simulink model "Single_phase_input_in_sine_Wave"  (R2021a)
settings: Solver=VariableStepAuto  StartTime=0.0  StopTime=1  RelTol=1e-3
undefined symbols (not defined in the file): Ion, Lithium
libraries: spsDiodeLib x8, spsVoltageMeasurementLib x7, spsSeriesRLCBranchLib x6, spsCurrentMeasurementLib x6, spsMosfetLib x4, spsACVoltageSourceLib x1, spsBatteryLib x1, spsImpedanceMeasurementLib x1, spsMutualInductanceLib x1, simulink x1, spspowerguiLib x1
settings Model: Creator=HP  LastModifiedBy=ADMIN

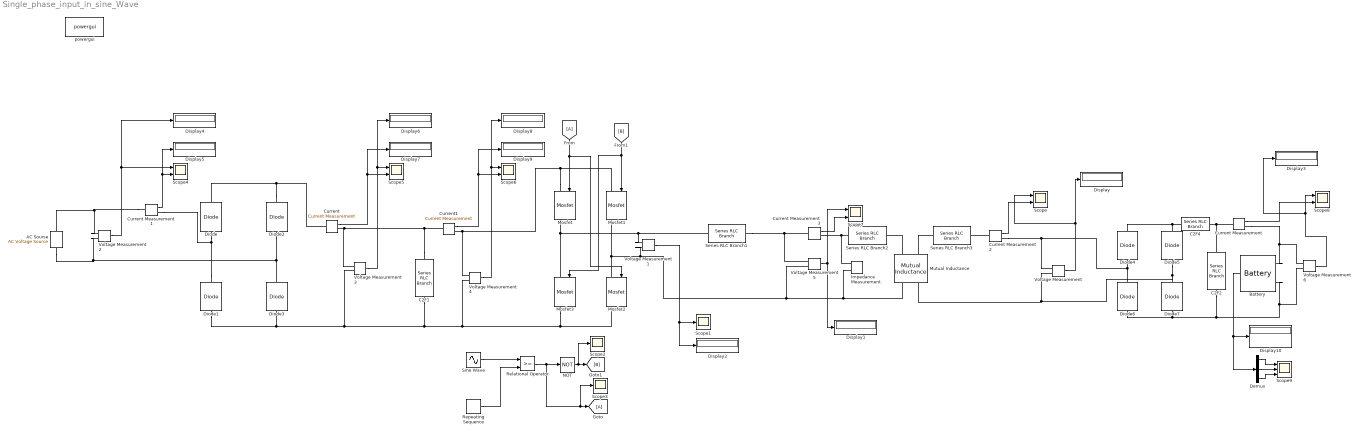
== system Single_phase_input_in_sine_Wave ==
  AC Sourse : spsACVoltageSourceLib/AC Voltage Source  Amplitude=325  Phase=0  Frequency=50  SampleTime=0  Measurements=Voltage  BusType=swing  Pref=10e3  Qref=0  Qmin=-inf  Qmax=+inf
  Battery : spsBatteryLib/Battery  BatType=Lithium-Ion  ShowTempParam=off  ThermalPreset=no  ShowAgeParam=off  NomV=240  NomQ=1  SOC=50  Batt_Tr=30  PresetModel=on  MaxQ=1  MinV=180  FullV=279.3569  Dis_rate=0.43478  R=2.4  Normal_OP=0.90435  expZone="[259.2926    0.04913043]"  current=[6.5 13 32.5]  Units=Time  Tci=20  NomT=20  T2=-30  MaxQ2=4.8  FullV2=7.1  Normal_OP2=5.655  expZone2="[6.58           1]"  Rca=0.6  ti=2000  Dp=0  Neq0=0  Tsim=1e6  Ta1=25  Qeol=5.4*0.9  Reol=0.013333*1.2  Char_age=[2.3478, 3]  Dis_age=[2.3478, 10]  N1=1500  N2=10500  N3=1000  N4=1400  Ta2=45  N5=950
  C2F1 : spsSeriesRLCBranchLib/Series RLC Branch  LConnTagsString=__new0  RConnTagsString=__new0  BranchType=C  Resistance=1e-6  Inductance=1e-3  SetiL0=off  InitialCurrent=0  Capacitance=300e-5  Setx0=off  InitialVoltage=0  Measurements=None
  C2F2 : spsSeriesRLCBranchLib/Series RLC Branch  LConnTagsString=__new0  RConnTagsString=__new0  BranchType=C  Resistance=1e-6  Inductance=1e-3  SetiL0=off  InitialCurrent=0  Capacitance=5e-6  Setx0=off  InitialVoltage=0  Measurements=None
  C2F4 : spsSeriesRLCBranchLib/Series RLC Branch  LConnTagsString=__new0  RConnTagsString=__new0  BranchType=L  Resistance=1e-6  Inductance=1e-6  SetiL0=off  InitialCurrent=0  Capacitance=5e-6  Setx0=off  InitialVoltage=0  Measurements=None
  Current : spsCurrentMeasurementLib/Current Measurement  PhasorSimulation=off  OutputType=Complex  PSBequivalent=0
  Current Measurement{,1..3} (4 alike) : spsCurrentMeasurementLib/Current Measurement  PhasorSimulation=off  OutputType=Complex  PSBequivalent=0
  Current1 : spsCurrentMeasurementLib/Current Measurement  PhasorSimulation=off  OutputType=Complex  PSBequivalent=0
  Demux : Demux  Outputs=3
  Diode{,1..7} (8 alike) : spsDiodeLib/Diode  Ron=0.001  Lon=0  Vf=0.8  IC=0  UseSnubber=0  Rs=500  Cs=250e-9  Measurements=off
  Display{,1..10} (11 alike) : Display
  Impedance Measurement : spsImpedanceMeasurementLib/Impedance Measurement  LConnTagsString=+|-  Factor=1
      settings: SourceProductBaseCode=PS
  Mosfet{,1..3} (4 alike) : spsMosfetLib/Mosfet  Ron=0.1  Lon=0  Rd=0.01  Vfd=0  IC=0  Rs=1e5  Cs=inf  Measurements=on
  Mutual Inductance : spsMutualInductanceLib/Mutual Inductance  LConnTagsString=a|b  RConnTagsString=A|B  TypeOfMutual=Two or three windings with equal mutual terms  NumberOfWindings=3  SelfImpedance1=[0.0714 73.43e-06]  SelfImpedance2=[0.0714 73.43e-06]  ThreeWindings=off  SelfImpedance3=[ 1.1 1.1e-03]  MutualImpedance=[0.01428 14.86e-06]  InductanceMatrix="[1.0 0.9  0.9 ;  0.9 1.0  0.9;  0.9 0.9 1.0 ] * 1e-3"  ResistanceMatrix="[1.0 0.9  0.9 ;  0.9 1.0  0.9;  0.9 0.9 1.0 ]"  Measurements=None
      settings: SourceProductBaseCode=PS
  NOT : Logic  Operator=NOT  IconShape=distinctive  AllPortsSameDT=off  OutDataTypeStr=boolean
  Relational Operator : RelationalOperator  OutDataTypeStr=boolean  RndMeth=Simplest
  Repeating Sequence : simulink/Sources/Repeating Sequence  rep_seq_t=[0 0.0000005 0.000001]  rep_seq_y=[-1 1 -1]
  Scope{,4..8} (6 alike) : Scope  NumInputPorts=2
  Scope1 : Scope
  Scope2 : Scope
  Scope3 : Scope
  Scope9 : Scope  NumInputPorts=3
  Series RLC Branch1 : spsSeriesRLCBranchLib/Series RLC Branch  LConnTagsString=__new0  RConnTagsString=__new0  BranchType=R  Resistance=2  Inductance=1e-3  SetiL0=off  InitialCurrent=0  Capacitance=34.5e-9  Setx0=off  InitialVoltage=0  Measurements=None
  Series RLC Branch2 : spsSeriesRLCBranchLib/Series RLC Branch  LConnTagsString=__new0  RConnTagsString=__new0  BranchType=C  Resistance=1  Inductance=1e-3  SetiL0=off  InitialCurrent=0  Capacitance=34.5e-9  Setx0=off  InitialVoltage=0  Measurements=None
  Series RLC Branch3 : spsSeriesRLCBranchLib/Series RLC Branch  LConnTagsString=__new0  RConnTagsString=__new0  BranchType=C  Resistance=1  Inductance=1e-3  SetiL0=off  InitialCurrent=0  Capacitance=34.5e-9  Setx0=off  InitialVoltage=0  Measurements=None
  Sine Wave : Sin  Amplitude=0.45  Frequency=2*pi*100000  SampleTime=0
  Voltage Measurement{,1..6} (7 alike) : spsVoltageMeasurementLib/Voltage Measurement  PhasorSimulation=off  OutputType=Complex  PSBequivalent=0
  powergui : spspowerguiLib/powergui  Priority=1  SimulationMode=Continuous  SampleTime=5e-7  frequency=60  Iterations=50  frequencyindice=0  Pbase=100e6  ErrMax=1e-4  UnitsV=kV  UnitsW=MW  buscounter=0  FunctionMessages=off  echomessages=off  EnableUseOfTLC=off  CurrentSourceSwitches=off  DisableSnubberDevices=off  DisableRonSwitches=off  DisableVfSwitches=off  DisplayEquations=off  AutomaticDiscreteSolvers=off  SolverType=Tustin/Backward Euler (TBE)  Interpol=off  ExternalGateDelay=off  methode=off  Ts=100  x0status=blocks  SPID=on  SwTol=0  HookPort=off  NonlinearTolerance=1e-4  nMaxIteration=100  ContinueOnMaxIteration=off  RestoreLinks=warning  ResistiveCurrentMeasurement=off  Frange=[0:2:1100000]  Ylog=on  Xlog=off  ShowGrid=off  save=off  variable=ZData  structure=0  ZoomFFT=off  StartTime=0.0  cycles=1  DisplayStyle=1  fundamental=60  FreqAxis=off  MaxFrequency=1000  frequencyindicesteady=1  RmsSteady=1  display=off
  wires:
  Voltage Measurement2/1 -> Scope4/1, Display4/1
  Voltage Measurement3/1 -> Scope5/1, Display6/1
  Sine Wave/1 -> Relational Operator/1
  Repeating Sequence/1 -> Relational Operator/2
  [A] -> Mosfet2/1, Mosfet/1
  NOT/1 -> Scope2/1, [B]
  Voltage Measurement6/1 -> Display3/1, Scope8/1
  Relational Operator/1 -> Scope3/1, [A], NOT/1
  Current Measurement/1 -> Scope8/2
  Voltage Measurement5/1 -> Scope7/1, Display1/1
  Current Measurement3/1 -> Scope7/2
  Current/1 -> Display7/1, Scope5/2
  Voltage Measurement4/1 -> Display8/1, Scope6/1
  Voltage Measurement/1 -> Display/1, Scope/1
  Current Measurement2/1 -> Scope/2
  Current Measurement1/1 -> Display5/1, Scope4/2
  Current1/1 -> Display9/1, Scope6/2
  Voltage Measurement1/1 -> Scope1/1, Display2/1
  [B] -> Mosfet3/1, Mosfet1/1
  Battery/1 -> Demux/1, Display10/1
  Demux/1 -> Scope9/1
  Demux/2 -> Scope9/2
  Demux/3 -> Scope9/3
  connections:
  Mosfet/LConn1 -- Current1/RConn1 -- Voltage Measurement4/LConn1 -- Mosfet1/LConn1
  Mosfet2/LConn1 -- Voltage Measurement5/LConn2 -- Impedance Measurement/LConn2 -- Mutual Inductance/RConn1 -- Voltage Measurement1/LConn2 -- Mosfet1/RConn1
  C2F4/RConn1 -- C2F2/LConn1 -- Current Measurement/LConn1
  Current Measurement/RConn1 -- Battery/LConn1 -- Voltage Measurement6/LConn1
  Diode5/RConn1 -- Diode4/RConn1 -- C2F4/LConn1
  C2F2/RConn1 -- Battery/LConn2 -- Voltage Measurement6/LConn2 -- Diode6/LConn1 -- Diode7/LConn1
  Voltage Measurement2/LConn2 -- AC Sourse/LConn1 -- Diode2/LConn1 -- Diode3/RConn1
  Series RLC Branch2/LConn1 -- Current Measurement3/RConn1 -- Impedance Measurement/LConn1
  Diode2/RConn1 -- Diode/RConn1 -- Current/LConn1
  C2F1/LConn1 -- Current/RConn1 -- Voltage Measurement3/LConn1 -- Current1/LConn1
  Current Measurement1/LConn1 -- AC Sourse/RConn1 -- Voltage Measurement2/LConn1
  Diode7/RConn1 -- Diode5/LConn1 -- Mutual Inductance/RConn2 -- Voltage Measurement/LConn2
  Current Measurement2/RConn1 -- Diode6/RConn1 -- Diode4/LConn1 -- Voltage Measurement/LConn1
  Diode1/RConn1 -- Diode/LConn1 -- Current Measurement1/RConn1
  Voltage Measurement1/LConn1 -- Series RLC Branch1/LConn1 -- Mosfet3/LConn1 -- Mosfet/RConn1
  C2F1/RConn1 -- Voltage Measurement4/LConn2 -- Mosfet2/RConn1 -- Mosfet3/RConn1 -- Voltage Measurement3/LConn2 -- Diode3/LConn1 -- Diode1/LConn1
  Current Measurement2/LConn1 -- Series RLC Branch3/RConn1
  Mutual Inductance/LConn2 -- Series RLC Branch3/LConn1
  Mutual Inductance/LConn1 -- Series RLC Branch2/RConn1
  Voltage Measurement5/LConn1 -- Current Measurement3/LConn1 -- Series RLC Branch1/RConn1
